simulink model "misurazione"  (R2021b)
settings: Solver=ode3  StartTime=0.0  StopTime=2  FixedStep=Ts  RelTol=1e-3
settings Model: Creator=antony  LastModifiedBy=antony

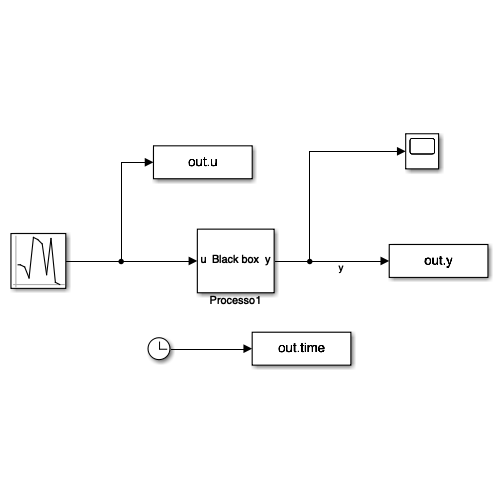
[thumbnail: Simulink's stored preview of the top-level diagram]
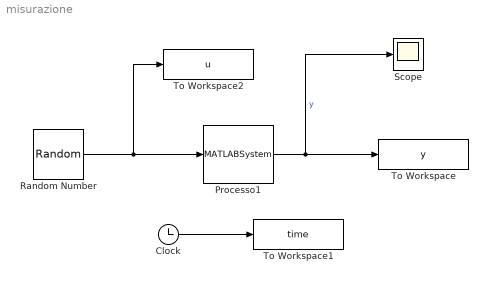
== system misurazione ==
  Clock : Clock
  Processo1 : MATLABSystem  System=linSysObj  SimulateUsing=Interpreted execution
      mask Type: linSysObj
      mask Display:
      | disp('Black box');
      | port_label('input',1,'u');
      | port_label('output',1,'y');
  Random Number : RandomNumber  SampleTime=0.01
  Scope : Scope
  To Workspace : ToWorkspace  VariableName=y  SampleTime=-1
      settings: Save2DSignal=2-D array (concatenate along first dimension)
  To Workspace1 : ToWorkspace  VariableName=time  SampleTime=-1
      settings: Save2DSignal=2-D array (concatenate along first dimension)
  To Workspace2 : ToWorkspace  VariableName=u  SampleTime=-1
      settings: Save2DSignal=2-D array (concatenate along first dimension)
  wires:
  Processo1/1 -> Scope/1, To Workspace/1  "y"
  Clock/1 -> To Workspace1/1
  Random Number/1 -> To Workspace2/1, Processo1/1
